simulink model "CF018A_GmRoadWhlInQlfr"  (R2013b)
settings: Solver=FixedStepDiscrete  SolverMode=SingleTasking  StartTime=0.0  StopTime=1  FixedStep=0.002  RelTol=1e-3
values from neighbouring files (symbols this model uses):
  DELTAPLSROLLOVR_CNT_S16 = DataDict.Constant    [CF018A_GmRoadWhlInQlfr_DataDict.m]
  DELTATISTAMPCNTROLLOVR_CNT_S32 = DataDict.Constant    [CF018A_GmRoadWhlInQlfr_DataDict.m]
  GmRoadWhlInQlfrMaxAllwblFrq = DataDict.Calibration    [CF018A_GmRoadWhlInQlfr_DataDict.m]
  GmRoadWhlInQlfrMaxFrqChg = DataDict.Calibration    [CF018A_GmRoadWhlInQlfr_DataDict.m]
  LEFRQCHGOUTOFRNG_CNT_U08 = DataDict.Constant    [CF018A_GmRoadWhlInQlfr_DataDict.m]
  LEFRQOUTOFRNG_CNT_U08 = DataDict.Constant    [CF018A_GmRoadWhlInQlfr_DataDict.m]
  NODEBSTEP_CNT_U16 = DataDict.Constant    [CF018A_GmRoadWhlInQlfr_DataDict.m]
  PARKDURN_CNT_F32 = DataDict.Constant    [CF018A_GmRoadWhlInQlfr_DataDict.m]
  PREVRAWWHLFRQMIN_HZ_F32 = DataDict.Constant    [CF018A_GmRoadWhlInQlfr_DataDict.m]
  RIFRQCHGOUTOFRNG_CNT_U08 = DataDict.Constant    [CF018A_GmRoadWhlInQlfr_DataDict.m]
  RIFRQOUTOFRNG_CNT_U08 = DataDict.Constant    [CF018A_GmRoadWhlInQlfr_DataDict.m]
  RoadWhlFrqInCalcOutOfRng = DataDict.NTC    [CF018A_GmRoadWhlInQlfr_DataDict.m]
  SECTO100MICROSECCNVN_CNT_F32 = DataDict.Constant    [CF018A_GmRoadWhlInQlfr_DataDict.m]
  WHLFRQMIN_HZ_F32 = DataDict.Constant    [CF018A_GmRoadWhlInQlfr_DataDict.m]
undefined symbols (not defined in the file or in its folder): NtcSts1
libraries: simulink x5, NxtrAbslt x2, NxtrLim x2
(part 4 of 5)

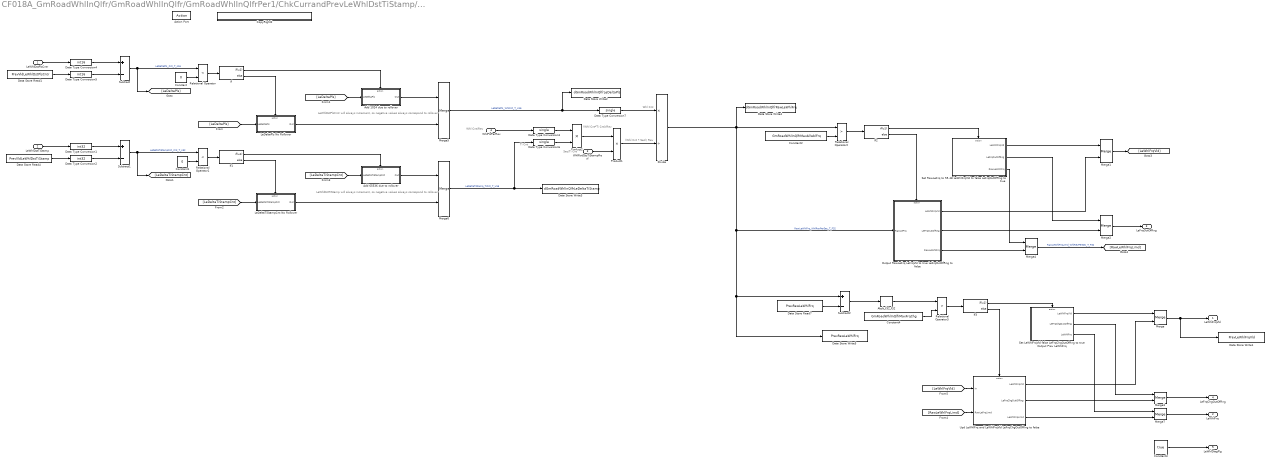
== system CF018A_GmRoadWhlInQlfr/GmRoadWhlInQlfr/GmRoadWhlInQlfrPer1/ChkCurrandPrevLeWhlDstTiStamp/Calc LeWhlFrq and LeWhlFrqVld /Calc LeWhlFrq and LeWhlFrqVld  ==
  note: Whl Cnt
  note: (Whl Cnt * Sec)/ Rev
  note: Ti Cnt
  note: Sec/Ti Cnt
  note: (Whl Cnt*Ti Cnt)/Rev
  note: Whl Cnt/Rev
  note: LeWhlDstTiStamp will always increment, so negative values always correspond to rollover
  note: LeWhlDstPlsCntr will always increment, so negative values always correspond to rollover
  LeWhlDstPlsCntr : Inport  RequirementInfo="{'linktype_rmi_doors' '0000c6e7 (/GM T1XX/SubSystem Specifications/Customer Functions/CF018A GM Road Wheel Input Qualifier)' '#170' 'true' 'REQ:  170' '' } %GIDa_81f6eb15_8b18_4642_a58d_cf70759d8f15"
  LeWhlDstTiStamp : Inport  RequirementInfo="{'linktype_rmi_doors' '0000c6e7 (/GM T1XX/SubSystem Specifications/Customer Functions/CF018A GM Road Wheel Input Qualifier)' '#170' 'true' 'REQ:  170' '' } %GIDa_7f9ec301_ef8f_4782_8c21_3364c3472735"  Port=2
  WhlRotlStsTiStampResl : Inport  RequirementInfo="{'linktype_rmi_doors' '0000c6e7 (/GM T1XX/SubSystem Specifications/Customer Functions/CF018A GM Road Wheel Input Qualifier)' '#170' 'true' 'REQ:  170' '' } %GIDa_d73dd23d_3d37_412a_b785_a9f4fffd0110"  Port=3
  WhlPlsPerRev : Inport  RequirementInfo="{'linktype_rmi_doors' '0000c6e7 (/GM T1XX/SubSystem Specifications/Customer Functions/CF018A GM Road Wheel Input Qualifier)' '#170' 'true' 'REQ:  170' '' } %GIDa_d298984b_0588_461a_81d7_4aff6f4fa4fc"  Port=4
  Action Port : ActionPort  ActionType=then
  Abslt_f32_f32 : NxtrAbslt/Abslt_f32_f32  RequirementInfo="{'linktype_rmi_doors' '0000c6e7 (/GM T1XX/SubSystem Specifications/Customer Functions/CF018A GM Road Wheel Input Qualifier)' '#176' 'true' 'REQ:  176' '' } %GIDa_9babf064_4138_43f4_bcce_3d87a0d45cc3"  SFunctionSpec=single y1 = Abslt_f32_f32(single u1)
      settings: AttributesFormatString=%<Name>
  Add 1024 due to rollover : Subsystem  RequirementInfo="{'linktype_rmi_doors' '0000c6e7 (/GM T1XX/SubSystem Specifications/Customer Functions/CF018A GM Road Wheel Input Qualifier)' '#170' 'true' 'REQ:  170' '' } %GIDa_49dd0180_17d4_41ca_993d_8e15b0be8cd1"  TreatAsAtomicUnit=on
  Add 65536 due to rollover : Subsystem  RequirementInfo="{'linktype_rmi_doors' '0000c6e7 (/GM T1XX/SubSystem Specifications/Customer Functions/CF018A GM Road Wheel Input Qualifier)' '#170' 'true' 'REQ:  170' '' } %GIDa_673682fc_2422_4a83_b510_e76deceeae94"  TreatAsAtomicUnit=on
  Constant : Constant  RequirementInfo="{'linktype_rmi_doors' '0000c6e7 (/GM T1XX/SubSystem Specifications/Customer Functions/CF018A GM Road Wheel Input Qualifier)' '#170' 'true' 'REQ:  170' '' } %GIDa_8b061d41_99c2_4522_a106_d56cc84f1816"  Value=0  OutDataTypeStr=int16
  Constant1 : Constant  RequirementInfo="{'linktype_rmi_doors' '0000c6e7 (/GM T1XX/SubSystem Specifications/Customer Functions/CF018A GM Road Wheel Input Qualifier)' '#170' 'true' 'REQ:  170' '' } %GIDa_ddec956e_1640_4ce9_b7f4_876fb629fee2"  Value=0  OutDataTypeStr=int32
  Constant2 : Constant  RequirementInfo="{'linktype_rmi_doors' '0000c6e7 (/GM T1XX/SubSystem Specifications/Customer Functions/CF018A GM Road Wheel Input Qualifier)' '#218' 'true' 'REQ:  218' '' ; 'linktype_rmi_doors' '0000c6e7 (/GM T1XX/SubSystem Specifications/Customer Functions/CF018A GM Road Wheel Input Qualifier)' '#175' 'true' 'REQ:  175' '' } %GIDa_4876d398_3911_425d_a27f_6993c3547bbd"  Value=GmRoadWhlInQlfrMaxAllwblFrq  OutDataTypeStr=single
  Constant3 : Constant  Value=true  OutDataTypeStr=boolean
      settings: AttributesFormatString=%<OutDataTypeStr>
  Constant4 : Constant  RequirementInfo="{'linktype_rmi_doors' '0000c6e7 (/GM T1XX/SubSystem Specifications/Customer Functions/CF018A GM Road Wheel Input Qualifier)' '#179' 'true' 'REQ:  179' '' ; 'linktype_rmi_doors' '0000c6e7 (/GM T1XX/SubSystem Specifications/Customer Functions/CF018A GM Road Wheel Input Qualifier)' '#176' 'true' 'REQ:  176' '' } %GIDa_f2aca31b_6717_44ff_958c_77a280e79e96"  Value=GmRoadWhlInQlfrMaxFrqChg
  CopyRight2 : Subsystem  Description=|  mask(Copyright Information){none=on}
      | Copyright info block.                                               
      |                                                                     
      | Place copyright information at the top of every subsystem in design.
      mask prompts: none "No parameters"
      mask help: Place copyright information at the top of every subsystem in design.
      mask Display:
      | NxtrConf = 'Nexteer Confidential';
      | 
      | sys = bdroot; %handle for the current model ("system")
      | first = get_param(sys,'Created');
      | if(isempty(first))
      |     first = datestr(now,'yyyy');
      | else
      |     first = first(end-3:end);  %year is last four digits
      | end
      | 
      | last = get_param(sys,'LastModifiedDate');
      | if isempty(last)
      |     last = datestr(now,'yyyy');
      | else
      |     last = last(end-3:end);
      | end
      | 
      | if strcmp(first,last)
      |     fprintf('%s -- Copyright %s Nexteer',NxtrConf,first)
      | else
      |     fprintf('%s -- %s%s- %s Nexteer',NxtrConf,char(169),first,last)
      | end
  Data Store Read1 : DataStoreRead  RequirementInfo="{'linktype_rmi_doors' '0000c6e7 (/GM T1XX/SubSystem Specifications/Customer Functions/CF018A GM Road Wheel Input Qualifier)' '#170' 'true' 'REQ:  170' '' } %GIDa_858aa324_7acc_4fd0_add3_db541b4b92e1"  DataStoreName=PrevVldLeWhlDstPlsCntr
  Data Store Read4 : DataStoreRead  RequirementInfo="{'linktype_rmi_doors' '0000c6e7 (/GM T1XX/SubSystem Specifications/Customer Functions/CF018A GM Road Wheel Input Qualifier)' '#170' 'true' 'REQ:  170' '' } %GIDa_7cd45e9a_58fd_4604_96cb_553a32710b34"  DataStoreName=PrevVldLeWhlDstTiStamp
  Data Store Read7 : DataStoreRead  RequirementInfo="{'linktype_rmi_doors' '0000c6e7 (/GM T1XX/SubSystem Specifications/Customer Functions/CF018A GM Road Wheel Input Qualifier)' '#176' 'true' 'REQ:  176' '' } %GIDa_a3115ec7_f18e_4431_ab97_984f5a4506dd"  Priority=0  DataStoreName=PrevRawLeWhlFrq
      settings: AttributesFormatString=%<Priority>
  Data Store Write1 : DataStoreWrite  RequirementInfo="{'linktype_rmi_doors' '0000c6e7 (/GM T1XX/SubSystem Specifications/Customer Functions/CF018A GM Road Wheel Input Qualifier)' '#176' 'true' 'REQ:  176' '' } %GIDa_ec08d42e_6251_41c8_b133_3f036ebc3510"  DataStoreName=PrevLeWhlFrqVld
      settings: AttributesFormatString=%<Priority>
  Data Store Write2 : DataStoreWrite  RequirementInfo="{'linktype_rmi_doors' '0000c6e7 (/GM T1XX/SubSystem Specifications/Customer Functions/CF018A GM Road Wheel Input Qualifier)' '#170' 'true' 'REQ:  170' '' } %GIDa_6506a920_d21b_4a41_8912_67910f5698ca"  DataStoreName=dGmRoadWhlInQlfrLeDeltaPls
  Data Store Write3 : DataStoreWrite  RequirementInfo="{'linktype_rmi_doors' '0000c6e7 (/GM T1XX/SubSystem Specifications/Customer Functions/CF018A GM Road Wheel Input Qualifier)' '#170' 'true' 'REQ:  170' '' } %GIDa_87548ccd_19bf_4323_b435_bb85d0142e2f"  DataStoreName=dGmRoadWhlInQlfrLeDeltaTiStamp
  Data Store Write4 : DataStoreWrite  RequirementInfo="{'linktype_rmi_doors' '0000c6e7 (/GM T1XX/SubSystem Specifications/Customer Functions/CF018A GM Road Wheel Input Qualifier)' '#175' 'true' 'REQ:  175' '' } %GIDa_013f3107_74ec_4409_b820_3123d1eae997"  DataStoreName=dGmRoadWhlInQlfrRawLeWhlFrq
  Data Store Write5 : DataStoreWrite  RequirementInfo="{'linktype_rmi_doors' '0000c6e7 (/GM T1XX/SubSystem Specifications/Customer Functions/CF018A GM Road Wheel Input Qualifier)' '#176' 'true' 'REQ:  176' '' } %GIDa_de1d07c8_712c_4036_8c18_78f028d520f4"  Priority=1  DataStoreName=PrevRawLeWhlFrq
      settings: AttributesFormatString=%<Priority>
  Data Type Conversion1 : DataTypeConversion  OutDataTypeStr=int32
  Data Type Conversion2 : DataTypeConversion  OutDataTypeStr=int32
  Data Type Conversion3 : DataTypeConversion  RequirementInfo="{'linktype_rmi_doors' '0000c6e7 (/GM T1XX/SubSystem Specifications/Customer Functions/CF018A GM Road Wheel Input Qualifier)' '#170' 'true' 'REQ:  170' '' } %GIDa_0b3a842d_d2aa_433d_8a7e_1a628cbde61e"  OutDataTypeStr=single
  Data Type Conversion4 : DataTypeConversion  OutDataTypeStr=int16
  Data Type Conversion5 : DataTypeConversion  OutDataTypeStr=int16
  Data Type Conversion6 : DataTypeConversion  RequirementInfo="{'linktype_rmi_doors' '0000c6e7 (/GM T1XX/SubSystem Specifications/Customer Functions/CF018A GM Road Wheel Input Qualifier)' '#170' 'true' 'REQ:  170' '' } %GIDa_d0f1bc26_581c_47ab_b06b_8b782c2ae32a"  OutDataTypeStr=single
  Data Type Conversion7 : DataTypeConversion  RequirementInfo="{'linktype_rmi_doors' '0000c6e7 (/GM T1XX/SubSystem Specifications/Customer Functions/CF018A GM Road Wheel Input Qualifier)' '#170' 'true' 'REQ:  170' '' } %GIDa_806b0f95_0ee7_4aef_8557_915ee92f77aa"  OutDataTypeStr=single
  Divide : Product  RequirementInfo="{'linktype_rmi_doors' '0000c6e7 (/GM T1XX/SubSystem Specifications/Customer Functions/CF018A GM Road Wheel Input Qualifier)' '#170' 'true' 'REQ:  170' '' } %GIDa_ecaab946_6f87_48de_9311_216db4035167"  Inputs=*/
      settings: AttributesFormatString=%<Priority>
  If : If  RequirementInfo="{'linktype_rmi_doors' '0000c6e7 (/GM T1XX/SubSystem Specifications/Customer Functions/CF018A GM Road Wheel Input Qualifier)' '#170' 'true' 'REQ:  170' '' } %GIDa_c1572c43_595f_4241_bfc8_833d91f05090"  IfExpression=u1
  If1 : If  RequirementInfo="{'linktype_rmi_doors' '0000c6e7 (/GM T1XX/SubSystem Specifications/Customer Functions/CF018A GM Road Wheel Input Qualifier)' '#170' 'true' 'REQ:  170' '' } %GIDa_8ea9250d_47f8_4248_b574_e8d129d6ab18"  IfExpression=u1
  If2 : If  RequirementInfo="{'linktype_rmi_doors' '0000c6e7 (/GM T1XX/SubSystem Specifications/Customer Functions/CF018A GM Road Wheel Input Qualifier)' '#175' 'true' 'REQ:  175' '' } %GIDa_3c20a0fd_f252_4d8c_93c2_0ab938042c19"  IfExpression=u1
  If3 : If  RequirementInfo="{'linktype_rmi_doors' '0000c6e7 (/GM T1XX/SubSystem Specifications/Customer Functions/CF018A GM Road Wheel Input Qualifier)' '#176' 'true' 'REQ:  176' '' } %GIDa_0bf69924_8eac_4bad_96f1_7da21f21de67"  IfExpression=u1
  LeDeltaPls No Rollover : Subsystem  RequirementInfo="{'linktype_rmi_doors' '0000c6e7 (/GM T1XX/SubSystem Specifications/Customer Functions/CF018A GM Road Wheel Input Qualifier)' '#170' 'true' 'REQ:  170' '' } %GIDa_731e1fb5_a310_441e_ab2e_f04067f21e71"  TreatAsAtomicUnit=on
  LeDeltaTiStampCnt No Rollover : Subsystem  RequirementInfo="{'linktype_rmi_doors' '0000c6e7 (/GM T1XX/SubSystem Specifications/Customer Functions/CF018A GM Road Wheel Input Qualifier)' '#170' 'true' 'REQ:  170' '' } %GIDa_baedfd9e_836e_480d_9447_1e736d4e0fac"  TreatAsAtomicUnit=on
  Merge : Merge  RequirementInfo="{'linktype_rmi_doors' '0000c6e7 (/GM T1XX/SubSystem Specifications/Customer Functions/CF018A GM Road Wheel Input Qualifier)' '#176' 'true' 'REQ:  176' '' } %GIDa_51a3869e_ea98_4a3c_8ce5_bfb21175d061"
  Merge1 : Merge  RequirementInfo="{'linktype_rmi_doors' '0000c6e7 (/GM T1XX/SubSystem Specifications/Customer Functions/CF018A GM Road Wheel Input Qualifier)' '#175' 'true' 'REQ:  175' '' } %GIDa_4ee51a38_6586_419f_8521_cb767c7b3f04"
  Merge2 : Merge  RequirementInfo="{'linktype_rmi_doors' '0000c6e7 (/GM T1XX/SubSystem Specifications/Customer Functions/CF018A GM Road Wheel Input Qualifier)' '#175' 'true' 'REQ:  175' '' } %GIDa_5e7a4cc5_3ac2_4b71_ba3d_f061c882e117"
  Merge3 : Merge  RequirementInfo="{'linktype_rmi_doors' '0000c6e7 (/GM T1XX/SubSystem Specifications/Customer Functions/CF018A GM Road Wheel Input Qualifier)' '#176' 'true' 'REQ:  176' '' } %GIDa_4213d823_ddd0_495b_8a3d_1c6b4d776feb"
  Merge4 : Merge  RequirementInfo="{'linktype_rmi_doors' '0000c6e7 (/GM T1XX/SubSystem Specifications/Customer Functions/CF018A GM Road Wheel Input Qualifier)' '#175' 'true' 'REQ:  175' '' } %GIDa_2a1d9456_a63f_4485_83e8_e75f4ada7506"
  Merge5 : Merge  RequirementInfo="{'linktype_rmi_doors' '0000c6e7 (/GM T1XX/SubSystem Specifications/Customer Functions/CF018A GM Road Wheel Input Qualifier)' '#170' 'true' 'REQ:  170' '' } %GIDa_5b3df2ac_8a4a_439d_a557_913bc624ef85"
  Merge6 : Merge  RequirementInfo="{'linktype_rmi_doors' '0000c6e7 (/GM T1XX/SubSystem Specifications/Customer Functions/CF018A GM Road Wheel Input Qualifier)' '#170' 'true' 'REQ:  170' '' } %GIDa_5feceb6f_cf07_4d53_9b7a_58b2e1e87157"
  Merge7 : Merge  RequirementInfo="{'linktype_rmi_doors' '0000c6e7 (/GM T1XX/SubSystem Specifications/Customer Functions/CF018A GM Road Wheel Input Qualifier)' '#176' 'true' 'REQ:  176' '' } %GIDa_158f11e6_aafd_45d3_bb19_68f95431a00e"
  Output RawLeFrq LeFrqVld to true LeFrqOutOfRng to false : Subsystem  RequirementInfo="{'linktype_rmi_doors' '0000c6e7 (/GM T1XX/SubSystem Specifications/Customer Functions/CF018A GM Road Wheel Input Qualifier)' '#175' 'true' 'REQ:  175' '' } %GIDa_de6b13e0_e9eb_4a05_8dff_8bfc345d5c25"  TreatAsAtomicUnit=on
  Product1 : Product  RequirementInfo="{'linktype_rmi_doors' '0000c6e7 (/GM T1XX/SubSystem Specifications/Customer Functions/CF018A GM Road Wheel Input Qualifier)' '#170' 'true' 'REQ:  170' '' } %GIDa_e290239d_3e19_4a86_aa29_128c5d82eca0"
  Product2 : Product  RequirementInfo="{'linktype_rmi_doors' '0000c6e7 (/GM T1XX/SubSystem Specifications/Customer Functions/CF018A GM Road Wheel Input Qualifier)' '#170' 'true' 'REQ:  170' '' } %GIDa_4677af3e_0b4c_43df_8a08_cd284f17272b"
  Relational Operator : RelationalOperator  RequirementInfo="{'linktype_rmi_doors' '0000c6e7 (/GM T1XX/SubSystem Specifications/Customer Functions/CF018A GM Road Wheel Input Qualifier)' '#170' 'true' 'REQ:  170' '' } %GIDa_752c2c9e_41d6_492c_850f_450902082c43"  Operator=<  OutDataTypeStr=boolean
  Relational Operator1 : RelationalOperator  RequirementInfo="{'linktype_rmi_doors' '0000c6e7 (/GM T1XX/SubSystem Specifications/Customer Functions/CF018A GM Road Wheel Input Qualifier)' '#170' 'true' 'REQ:  170' '' } %GIDa_f32f7a75_e353_422e_832d_c9335738dc5a"  Operator=<  OutDataTypeStr=boolean
  Relational Operator2 : RelationalOperator  RequirementInfo="{'linktype_rmi_doors' '0000c6e7 (/GM T1XX/SubSystem Specifications/Customer Functions/CF018A GM Road Wheel Input Qualifier)' '#175' 'true' 'REQ:  175' '' } %GIDa_a36d66af_8ed3_4599_8ceb_4e44b369b520"  Operator=>  OutDataTypeStr=boolean
  Relational Operator3 : RelationalOperator  RequirementInfo="{'linktype_rmi_doors' '0000c6e7 (/GM T1XX/SubSystem Specifications/Customer Functions/CF018A GM Road Wheel Input Qualifier)' '#176' 'true' 'REQ:  176' '' } %GIDa_280c3b32_0b0f_4faa_b9b8_ef69c1361a72"  Operator=>  OutDataTypeStr=boolean
  Set LeWhlFrqVld false LeFrqChgOutOfRng to true Output Prev LeWhlFrq : Subsystem  RequirementInfo="{'linktype_rmi_doors' '0000c6e7 (/GM T1XX/SubSystem Specifications/Customer Functions/CF018A GM Road Wheel Input Qualifier)' '#176' 'true' 'REQ:  176' '' } %GIDa_69e17394_4547_4791_9f0a_6f0549775007"  TreatAsAtomicUnit=on
  Set RawLeFrq to 55.48 LeWhlFrqVld to false LeFrqOutOfRng to true : Subsystem  RequirementInfo="{'linktype_rmi_doors' '0000c6e7 (/GM T1XX/SubSystem Specifications/Customer Functions/CF018A GM Road Wheel Input Qualifier)' '#175' 'true' 'REQ:  175' '' } %GIDa_ca636fc7_8999_459a_8a1a_72b0b121a43f"  TreatAsAtomicUnit=on
  Subtract : Sum  RequirementInfo="{'linktype_rmi_doors' '0000c6e7 (/GM T1XX/SubSystem Specifications/Customer Functions/CF018A GM Road Wheel Input Qualifier)' '#170' 'true' 'REQ:  170' '' } %GIDa_a619972a_c82a_4aa5_8379_e381c0276a01"  Inputs=+-  OutDataTypeStr=int16
      settings: AttributesFormatString=%<Priority>
  Subtract1 : Sum  RequirementInfo="{'linktype_rmi_doors' '0000c6e7 (/GM T1XX/SubSystem Specifications/Customer Functions/CF018A GM Road Wheel Input Qualifier)' '#170' 'true' 'REQ:  170' '' } %GIDa_988c2c08_2083_452e_80ea_7c9ead94b42f"  Inputs=+-  OutDataTypeStr=int32
      settings: AttributesFormatString=%<Priority>
  Subtract2 : Sum  RequirementInfo="{'linktype_rmi_doors' '0000c6e7 (/GM T1XX/SubSystem Specifications/Customer Functions/CF018A GM Road Wheel Input Qualifier)' '#176' 'true' 'REQ:  176' '' } %GIDa_824b8546_ee4a_4296_8369_853dd7941f8a"  Inputs=+-
  Upd LeWhlFrq and LeWhlFrqVld LeFrqChgOutOfRng to false : Subsystem  RequirementInfo="{'linktype_rmi_doors' '0000c6e7 (/GM T1XX/SubSystem Specifications/Customer Functions/CF018A GM Road Wheel Input Qualifier)' '#176' 'true' 'REQ:  176' '' } %GIDa_d364e30d_9bb3_46d4_87ee_ef84be4eddae"  TreatAsAtomicUnit=on
  LeWhlFrqVld : Outport  RequirementInfo="{'linktype_rmi_doors' '0000c6e7 (/GM T1XX/SubSystem Specifications/Customer Functions/CF018A GM Road Wheel Input Qualifier)' '#176' 'true' 'REQ:  176' '' } %GIDa_bf05f879_8f7d_42a0_b324_aeb1286c9553"
  LeWhlFrq : Outport  RequirementInfo="{'linktype_rmi_doors' '0000c6e7 (/GM T1XX/SubSystem Specifications/Customer Functions/CF018A GM Road Wheel Input Qualifier)' '#176' 'true' 'REQ:  176' '' } %GIDa_d83b31f1_6e5b_4863_aa9e_369246e7f69e"  Port=2
  LeFrqOutOfRng : Outport  RequirementInfo="{'linktype_rmi_doors' '0000c6e7 (/GM T1XX/SubSystem Specifications/Customer Functions/CF018A GM Road Wheel Input Qualifier)' '#175' 'true' 'REQ:  175' '' } %GIDa_69a60709_30d0_4c0e_afbd_b91f3e065487"  Port=3
  LeFrqChgOutOfRng : Outport  RequirementInfo="{'linktype_rmi_doors' '0000c6e7 (/GM T1XX/SubSystem Specifications/Customer Functions/CF018A GM Road Wheel Input Qualifier)' '#176' 'true' 'REQ:  176' '' } %GIDa_3d57b922_5289_402f_9db8_c179b75ec954"  Port=4
  LeWhlDiagFlg : Outport  Port=5
  wires:
  If/1 -> Add 1024 due to rollover/Action
  LeWhlDstPlsCntr/1 -> Data Type Conversion4/1
  Subtract/1 -> [LeDeltaPls], Relational Operator/1  "LeDeltaPls_Cnt_T_s16"
  Relational Operator/1 -> If/1
  Constant/1 -> Relational Operator/2
  If1/1 -> Add 65536 due to rollover/Action
  Subtract1/1 -> [LeDeltaTiStampCnt], Relational Operator1/1  "LeDeltaTiStampCnt_Cnt_T_s32"
  Relational Operator1/1 -> If1/1
  Constant1/1 -> Relational Operator1/2
  Constant2/1 -> Relational Operator2/2
  Relational Operator2/1 -> If2/1
  If2/1 -> Set RawLeFrq to 55.48 LeWhlFrqVld to false LeFrqOutOfRng to true/Action
  Divide/1 -> Data Store Write4/1, Relational Operator2/1, Output RawLeFrq LeFrqVld to true LeFrqOutOfRng to false/1(RawLeFrq), Subtract2/1, Data Store Write5/1  "RawLeWhlFrq_WhlRevPerSec_T_F32"
  Data Store Read7/1 -> Subtract2/2
  Constant4/1 -> Relational Operator3/2
  Relational Operator3/1 -> If3/1
  Subtract2/1 -> Abslt_f32_f32/1
  If3/1 -> Set LeWhlFrqVld false LeFrqChgOutOfRng to true Output Prev LeWhlFrq/Action
  If3/2 -> Upd LeWhlFrq and LeWhlFrqVld LeFrqChgOutOfRng to false/Action
  Upd LeWhlFrq and LeWhlFrqVld LeFrqChgOutOfRng to false/1(LeWhlFrqVld) -> Merge/2
  Set LeWhlFrqVld false LeFrqChgOutOfRng to true Output Prev LeWhlFrq/1(LeWhlFrqVld) -> Merge/1
  Merge/1 -> Data Store Write1/1, LeWhlFrqVld/1
  If2/2 -> Output RawLeFrq LeFrqVld to true LeFrqOutOfRng to false/Action
  WhlPlsPerRev/1 -> Data Type Conversion3/1
  Abslt_f32_f32/1 -> Relational Operator3/1
  WhlRotlStsTiStampResl/1 -> Product1/2
  Product1/1 -> Divide/2
  [LeDeltaPls] -> LeDeltaPls No Rollover/1(LeDeltaPls)
  [LeDeltaTiStampCnt] -> LeDeltaTiStampCnt No Rollover/1(LeDeltaTiStampCnt)
  If/2 -> LeDeltaPls No Rollover/Action
  [LeDeltaPls] -> Add 1024 due to rollover/1(LeDeltaPls)
  If1/2 -> LeDeltaTiStampCnt No Rollover/Action
  [LeDeltaTiStampCnt] -> Add 65536 due to rollover/1(LeDeltaTiStampCnt)
  Product2/1 -> Product1/1
  Data Store Read1/1 -> Data Type Conversion5/1
  Data Type Conversion7/1 -> Divide/1
  Set RawLeFrq to 55.48 LeWhlFrqVld to false LeFrqOutOfRng to true/1(LeWhlFrqVld) -> Merge1/1
  Output RawLeFrq LeFrqVld to true LeFrqOutOfRng to false/1(LeWhlFrqVld) -> Merge1/2
  Merge2/1 -> LeFrqOutOfRng/1
  Set RawLeFrq to 55.48 LeWhlFrqVld to false LeFrqOutOfRng to true/2(LeFrqOutOfRng) -> Merge2/1
  Output RawLeFrq LeFrqVld to true LeFrqOutOfRng to false/2(LeFrqOutOfRng) -> Merge2/2
  [RawLeWhlFrqLimd] -> Upd LeWhlFrq and LeWhlFrqVld LeFrqChgOutOfRng to false/2(RawLeFrqLimd)
  Merge1/1 -> [LeWhlFrqVld]
  [LeWhlFrqVld] -> Upd LeWhlFrq and LeWhlFrqVld LeFrqChgOutOfRng to false/1(In)
  Set LeWhlFrqVld false LeFrqChgOutOfRng to true Output Prev LeWhlFrq/2(LeFrqChgOutOfRng) -> Merge3/1
  Merge3/1 -> LeFrqChgOutOfRng/1
  Output RawLeFrq LeFrqVld to true LeFrqOutOfRng to false/3(RawLeWhlFrq) -> Merge4/2
  Set RawLeFrq to 55.48 LeWhlFrqVld to false LeFrqOutOfRng to true/3(RawLeWhlFrq) -> Merge4/1
  Merge4/1 -> [RawLeWhlFrqLimd]  "RawLeWhlFrqLimd_WhlRevPerSec_T_F32"
  Upd LeWhlFrq and LeWhlFrqVld LeFrqChgOutOfRng to false/2(LeFrqChgOutOfRng) -> Merge3/2
  Add 1024 due to rollover/1(Out) -> Merge5/1
  LeDeltaPls No Rollover/1(Out) -> Merge5/2
  Merge5/1 -> Data Type Conversion7/1, Data Store Write2/1  "LeDeltaPls_WhlCnt_T_U16"
  Add 65536 due to rollover/1(Out) -> Merge6/1
  LeDeltaTiStampCnt No Rollover/1(Out) -> Merge6/2
  Merge6/1 -> Data Type Conversion6/1, Data Store Write3/1  "LeDeltaTiStamp_TiCnt_T_U16"
  Constant3/1 -> LeWhlDiagFlg/1
  Merge7/1 -> LeWhlFrq/1
  Set LeWhlFrqVld false LeFrqChgOutOfRng to true Output Prev LeWhlFrq/3(LeWhlFrq) -> Merge7/1
  Upd LeWhlFrq and LeWhlFrqVld LeFrqChgOutOfRng to false/3(LeWhlFrqLimd) -> Merge7/2
  LeWhlDstTiStamp/1 -> Data Type Conversion1/1
  Data Store Read4/1 -> Data Type Conversion2/1
  Data Type Conversion2/1 -> Subtract1/2
  Data Type Conversion1/1 -> Subtract1/1
  Data Type Conversion6/1 -> Product2/2
  Data Type Conversion5/1 -> Subtract/2
  Data Type Conversion4/1 -> Subtract/1
  Data Type Conversion3/1 -> Product2/1

== system CF018A_GmRoadWhlInQlfr/GmRoadWhlInQlfr/GmRoadWhlInQlfrPer1/ChkCurrandPrevLeWhlDstTiStamp/Calc LeWhlFrq and LeWhlFrqVld /CopyRight2 ==

== system CF018A_GmRoadWhlInQlfr/GmRoadWhlInQlfr/GmRoadWhlInQlfrPer1/ChkCurrandPrevLeWhlDstTiStamp/Calc LeWhlFrq and LeWhlFrqVld /GetRefTmr100MicroSec32bit ==
  note: 1 count = 100 uSec
  note: seconds
  note: microseconds
  note: counts
  note: Wrap-to-zero
  note: GetRefTmr100MicroSec32bit
  note: Created Aug 18, 2015
      | Modified Oct 21, 2015
      | Modified Oct 30, 2015
      | Kevin Derry
  CopyRight2 : Subsystem  Description=|  mask(Copyright Information){none=on}
      | Copyright info block.                                               
      |                                                                     
      | Place copyright information at the top of every subsystem in design.
      mask prompts: none "No parameters"
      mask help: Place copyright information at the top of every subsystem in design.
      mask Display:
      | NxtrConf = 'Nexteer Confidential';
      | 
      | sys = bdroot; %handle for the current model ("system")
      | first = get_param(sys,'Created');
      | if(isempty(first))
      |     first = datestr(now,'yyyy');
      | else
      |     first = first(end-3:end);  %year is last four digits
      | end
      | 
      | last = get_param(sys,'LastModifiedDate');
      | if isempty(last)
      |     last = datestr(now,'yyyy');
      | else
      |     last = last(end-3:end);
      | end
      | 
      | if strcmp(first,last)
      |     fprintf('%s -- Copyright %s Nexteer',NxtrConf,first)
      | else
      |     fprintf('%s -- %s%s- %s Nexteer',NxtrConf,char(169),first,last)
      | end
  Count per uSec : Constant  Value=0.01
  Data Store Read1 : DataStoreRead  DataStoreName=SimnTi
  Data Type Conversion1 : DataTypeConversion  OutDataTypeStr=uint32
  Divide1 : Product  Inputs=**
  Divide2 : Product  Inputs=*/
  Max Counts : Constant  Value=2^32-1
  Product1 : Product
  Product2 : Product
  Rounding : Rounding
  Subtract1 : Sum  Inputs=+-
  uSec per Sec : Constant  Value=1000000
  RefTmr : Outport
  wires:
  Product2/1 -> Subtract1/2
  Subtract1/1 -> Data Type Conversion1/1
  Rounding/1 -> Product2/1
  Divide2/1 -> Rounding/1
  Max Counts/1 -> Divide2/2, Product2/2
  Divide1/1 -> Divide2/1, Subtract1/1
  Product1/1 -> Divide1/1
  Count per uSec/1 -> Divide1/2
  uSec per Sec/1 -> Product1/2
  Data Type Conversion1/1 -> RefTmr/1
  Data Store Read1/1 -> Product1/1

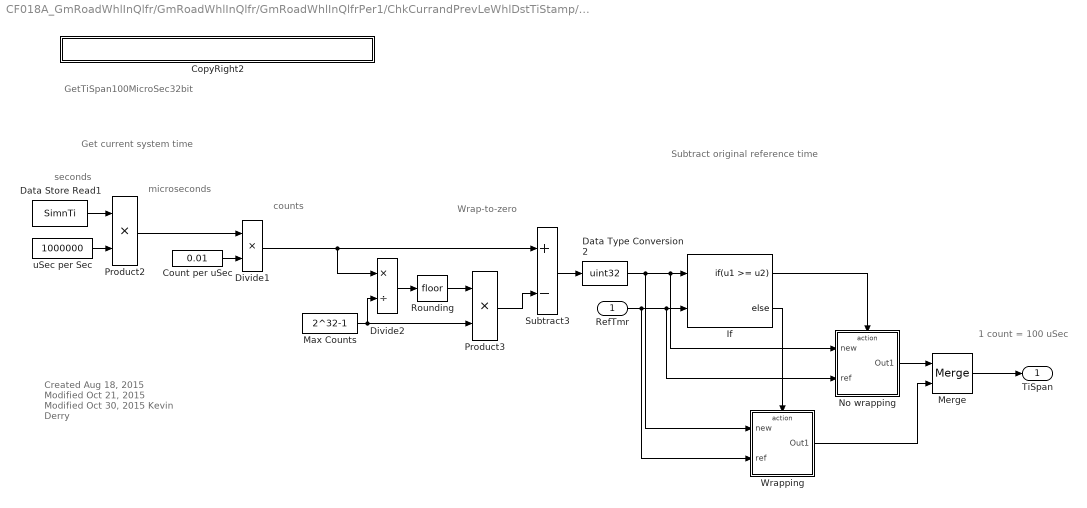
== system CF018A_GmRoadWhlInQlfr/GmRoadWhlInQlfr/GmRoadWhlInQlfrPer1/ChkCurrandPrevLeWhlDstTiStamp/Calc LeWhlFrq and LeWhlFrqVld /GetTiSpan100MicroSec32bit ==
  note: Created Aug 18, 2015
      | Modified Oct 21, 2015
      | Modified Oct 30, 2015
      | Kevin Derry
  note: GetTiSpan100MicroSec32bit
  note: Get current system time
  note: 1 count = 100 uSec
  note: Wrap-to-zero
  note: counts
  note: microseconds
  note: seconds
  note: Subtract original reference time
  RefTmr : Inport
  CopyRight2 : Subsystem  Description=|  mask(Copyright Information){none=on}
      | Copyright info block.                                               
      |                                                                     
      | Place copyright information at the top of every subsystem in design.
      mask prompts: none "No parameters"
      mask help: Place copyright information at the top of every subsystem in design.
      mask Display:
      | NxtrConf = 'Nexteer Confidential';
      | 
      | sys = bdroot; %handle for the current model ("system")
      | first = get_param(sys,'Created');
      | if(isempty(first))
      |     first = datestr(now,'yyyy');
      | else
      |     first = first(end-3:end);  %year is last four digits
      | end
      | 
      | last = get_param(sys,'LastModifiedDate');
      | if isempty(last)
      |     last = datestr(now,'yyyy');
      | else
      |     last = last(end-3:end);
      | end
      | 
      | if strcmp(first,last)
      |     fprintf('%s -- Copyright %s Nexteer',NxtrConf,first)
      | else
      |     fprintf('%s -- %s%s- %s Nexteer',NxtrConf,char(169),first,last)
      | end
  Count per uSec : Constant  Value=0.01
  Data Store Read1 : DataStoreRead  DataStoreName=SimnTi
  Data Type Conversion2 : DataTypeConversion  OutDataTypeStr=uint32
  Divide1 : Product  Inputs=**
  Divide2 : Product  Inputs=*/
  If : If  NumInputs=2  IfExpression=u1 >= u2
  Max Counts : Constant  Value=2^32-1
  Merge : Merge
  No wrapping : Subsystem  TreatAsAtomicUnit=on
  Product2 : Product
  Product3 : Product
  Rounding : Rounding
  Subtract3 : Sum  Inputs=+-
  Wrapping : Subsystem  TreatAsAtomicUnit=on
  uSec per Sec : Constant  Value=1000000
  TiSpan : Outport
  wires:
  Data Type Conversion2/1 -> Wrapping/1(new), No wrapping/1(new), If/1
  RefTmr/1 -> Wrapping/2(ref), No wrapping/2(ref), If/2
  Merge/1 -> TiSpan/1
  uSec per Sec/1 -> Product2/2
  Count per uSec/1 -> Divide1/2
  Data Store Read1/1 -> Product2/1
  Product2/1 -> Divide1/1
  Divide1/1 -> Subtract3/1, Divide2/1
  Max Counts/1 -> Product3/2, Divide2/2
  Divide2/1 -> Rounding/1
  Rounding/1 -> Product3/1
  Subtract3/1 -> Data Type Conversion2/1
  Product3/1 -> Subtract3/2
  If/1 -> No wrapping/Action
  If/2 -> Wrapping/Action
  No wrapping/1(Out1) -> Merge/1
  Wrapping/1(Out1) -> Merge/2

== system CF018A_GmRoadWhlInQlfr/GmRoadWhlInQlfr/GmRoadWhlInQlfrPer1/ChkCurrandPrevLeWhlDstTiStamp/Calc LeWhlFrq and LeWhlFrqVld /Prev LeWhlFrq and LeWhlFrqVld LeFrqOutOfRng to false LeFrqChgOutOfRng to false LeWhlDiagFlg to false  ==
  Action Port : ActionPort  ActionType=else
  Constant1 : Constant  Value=false  OutDataTypeStr=boolean
      settings: AttributesFormatString=%<OutDataTypeStr>
  Constant2 : Constant  Value=false  OutDataTypeStr=boolean
      settings: AttributesFormatString=%<OutDataTypeStr>
  Constant3 : Constant  Value=false  OutDataTypeStr=boolean
      settings: AttributesFormatString=%<OutDataTypeStr>
  CopyRight2 : Subsystem  Description=|  mask(Copyright Information){none=on}
      | Copyright info block.                                               
      |                                                                     
      | Place copyright information at the top of every subsystem in design.
      mask prompts: none "No parameters"
      mask help: Place copyright information at the top of every subsystem in design.
      mask Display:
      | NxtrConf = 'Nexteer Confidential';
      | 
      | sys = bdroot; %handle for the current model ("system")
      | first = get_param(sys,'Created');
      | if(isempty(first))
      |     first = datestr(now,'yyyy');
      | else
      |     first = first(end-3:end);  %year is last four digits
      | end
      | 
      | last = get_param(sys,'LastModifiedDate');
      | if isempty(last)
      |     last = datestr(now,'yyyy');
      | else
      |     last = last(end-3:end);
      | end
      | 
      | if strcmp(first,last)
      |     fprintf('%s -- Copyright %s Nexteer',NxtrConf,first)
      | else
      |     fprintf('%s -- %s%s- %s Nexteer',NxtrConf,char(169),first,last)
      | end
  Data Store Read2 : DataStoreRead  DataStoreName=PrevLeWhlFrqVld
      settings: AttributesFormatString=%<Priority>
  Data Store Read3 : DataStoreRead  DataStoreName=PrevLeWhlFrq
      settings: AttributesFormatString=%<Priority>
  LeWhlFrqVld : Outport
  LeWhlFrq : Outport  Port=2
  LeFrqOutOfRng : Outport  Port=3
  LeFrqChgOutOfRng : Outport  Port=4
  LeWhlDiagFlg : Outport  Port=5
  wires:
  Constant1/1 -> LeFrqOutOfRng/1
  Constant2/1 -> LeFrqChgOutOfRng/1
  Data Store Read2/1 -> LeWhlFrqVld/1
  Data Store Read3/1 -> LeWhlFrq/1
  Constant3/1 -> LeWhlDiagFlg/1

== system CF018A_GmRoadWhlInQlfr/GmRoadWhlInQlfr/GmRoadWhlInQlfrPer1/ChkCurrandPrevLeWhlDstTiStamp/Prev LeWhlFrq and LeWhlFrqVld LeFrqOutOfRng to false LeFrqChgOutOfRng to fasse LeWhlDiagFlg to false /CopyRight2 ==

== system CF018A_GmRoadWhlInQlfr/GmRoadWhlInQlfr/GmRoadWhlInQlfrPer1/NTC Diag/NTC 0x0E3 Faild/Bit0Sts fail ==
  Action Port : ActionPort  ActionType=then
  Constant : Constant  Value=LEFRQOUTOFRNG_CNT_U08
  CopyRight2 : Subsystem  Description=|  mask(Copyright Information){none=on}
      | Copyright info block.                                               
      |                                                                     
      | Place copyright information at the top of every subsystem in design.
      mask prompts: none "No parameters"
      mask help: Place copyright information at the top of every subsystem in design.
      mask Display:
      | NxtrConf = 'Nexteer Confidential';
      | 
      | sys = bdroot; %handle for the current model ("system")
      | first = get_param(sys,'Created');
      | if(isempty(first))
      |     first = datestr(now,'yyyy');
      | else
      |     first = first(end-3:end);  %year is last four digits
      | end
      | 
      | last = get_param(sys,'LastModifiedDate');
      | if isempty(last)
      |     last = datestr(now,'yyyy');
      | else
      |     last = last(end-3:end);
      | end
      | 
      | if strcmp(first,last)
      |     fprintf('%s -- Copyright %s Nexteer',NxtrConf,first)
      | else
      |     fprintf('%s -- %s%s- %s Nexteer',NxtrConf,char(169),first,last)
      | end
  Bit0Sts : Outport
  wires:
  Constant/1 -> Bit0Sts/1

== system CF018A_GmRoadWhlInQlfr/GmRoadWhlInQlfr/GmRoadWhlInQlfrPer1/NTC Diag/NTC 0x0E3 Faild/Bit0Sts pass ==
  Action Port : ActionPort  ActionType=else
  Constant1 : Constant  Value=0  OutDataTypeStr=uint8
      settings: AttributesFormatString=%<OutDataTypeStr>
  CopyRight2 : Subsystem  Description=|  mask(Copyright Information){none=on}
      | Copyright info block.                                               
      |                                                                     
      | Place copyright information at the top of every subsystem in design.
      mask prompts: none "No parameters"
      mask help: Place copyright information at the top of every subsystem in design.
      mask Display:
      | NxtrConf = 'Nexteer Confidential';
      | 
      | sys = bdroot; %handle for the current model ("system")
      | first = get_param(sys,'Created');
      | if(isempty(first))
      |     first = datestr(now,'yyyy');
      | else
      |     first = first(end-3:end);  %year is last four digits
      | end
      | 
      | last = get_param(sys,'LastModifiedDate');
      | if isempty(last)
      |     last = datestr(now,'yyyy');
      | else
      |     last = last(end-3:end);
      | end
      | 
      | if strcmp(first,last)
      |     fprintf('%s -- Copyright %s Nexteer',NxtrConf,first)
      | else
      |     fprintf('%s -- %s%s- %s Nexteer',NxtrConf,char(169),first,last)
      | end
  Bit0Sts : Outport
  wires:
  Constant1/1 -> Bit0Sts/1

== system CF018A_GmRoadWhlInQlfr/GmRoadWhlInQlfr/GmRoadWhlInQlfrPer1/NTC Diag/NTC 0x0E3 Faild/Bit1Sts fail ==
  Action Port : ActionPort  ActionType=then
  Constant : Constant  Value=LEFRQCHGOUTOFRNG_CNT_U08
  CopyRight2 : Subsystem  Description=|  mask(Copyright Information){none=on}
      | Copyright info block.                                               
      |                                                                     
      | Place copyright information at the top of every subsystem in design.
      mask prompts: none "No parameters"
      mask help: Place copyright information at the top of every subsystem in design.
      mask Display:
      | NxtrConf = 'Nexteer Confidential';
      | 
      | sys = bdroot; %handle for the current model ("system")
      | first = get_param(sys,'Created');
      | if(isempty(first))
      |     first = datestr(now,'yyyy');
      | else
      |     first = first(end-3:end);  %year is last four digits
      | end
      | 
      | last = get_param(sys,'LastModifiedDate');
      | if isempty(last)
      |     last = datestr(now,'yyyy');
      | else
      |     last = last(end-3:end);
      | end
      | 
      | if strcmp(first,last)
      |     fprintf('%s -- Copyright %s Nexteer',NxtrConf,first)
      | else
      |     fprintf('%s -- %s%s- %s Nexteer',NxtrConf,char(169),first,last)
      | end
  Bit1Sts : Outport
  wires:
  Constant/1 -> Bit1Sts/1

== system CF018A_GmRoadWhlInQlfr/GmRoadWhlInQlfr/GmRoadWhlInQlfrPer1/NTC Diag/NTC 0x0E3 Faild/Bit1Sts pass ==
  Action Port : ActionPort  ActionType=else
  Constant1 : Constant  Value=0  OutDataTypeStr=uint8
      settings: AttributesFormatString=%<OutDataTypeStr>
  CopyRight2 : Subsystem  Description=|  mask(Copyright Information){none=on}
      | Copyright info block.                                               
      |                                                                     
      | Place copyright information at the top of every subsystem in design.
      mask prompts: none "No parameters"
      mask help: Place copyright information at the top of every subsystem in design.
      mask Display:
      | NxtrConf = 'Nexteer Confidential';
      | 
      | sys = bdroot; %handle for the current model ("system")
      | first = get_param(sys,'Created');
      | if(isempty(first))
      |     first = datestr(now,'yyyy');
      | else
      |     first = first(end-3:end);  %year is last four digits
      | end
      | 
      | last = get_param(sys,'LastModifiedDate');
      | if isempty(last)
      |     last = datestr(now,'yyyy');
      | else
      |     last = last(end-3:end);
      | end
      | 
      | if strcmp(first,last)
      |     fprintf('%s -- Copyright %s Nexteer',NxtrConf,first)
      | else
      |     fprintf('%s -- %s%s- %s Nexteer',NxtrConf,char(169),first,last)
      | end
  Bit1Sts : Outport
  wires:
  Constant1/1 -> Bit1Sts/1

== system CF018A_GmRoadWhlInQlfr/GmRoadWhlInQlfr/GmRoadWhlInQlfrPer1/NTC Diag/NTC 0x0E3 Faild/Bit4Sts fail ==
  Action Port : ActionPort  ActionType=then
  Constant : Constant  Value=RIFRQOUTOFRNG_CNT_U08
  CopyRight2 : Subsystem  Description=|  mask(Copyright Information){none=on}
      | Copyright info block.                                               
      |                                                                     
      | Place copyright information at the top of every subsystem in design.
      mask prompts: none "No parameters"
      mask help: Place copyright information at the top of every subsystem in design.
      mask Display:
      | NxtrConf = 'Nexteer Confidential';
      | 
      | sys = bdroot; %handle for the current model ("system")
      | first = get_param(sys,'Created');
      | if(isempty(first))
      |     first = datestr(now,'yyyy');
      | else
      |     first = first(end-3:end);  %year is last four digits
      | end
      | 
      | last = get_param(sys,'LastModifiedDate');
      | if isempty(last)
      |     last = datestr(now,'yyyy');
      | else
      |     last = last(end-3:end);
      | end
      | 
      | if strcmp(first,last)
      |     fprintf('%s -- Copyright %s Nexteer',NxtrConf,first)
      | else
      |     fprintf('%s -- %s%s- %s Nexteer',NxtrConf,char(169),first,last)
      | end
  Bit0Sts : Outport
  wires:
  Constant/1 -> Bit0Sts/1

== system CF018A_GmRoadWhlInQlfr/GmRoadWhlInQlfr/GmRoadWhlInQlfrPer1/NTC Diag/NTC 0x0E3 Faild/Bit4Sts pass ==
  Action Port : ActionPort  ActionType=else
  Constant1 : Constant  Value=0  OutDataTypeStr=uint8
      settings: AttributesFormatString=%<OutDataTypeStr>
  CopyRight2 : Subsystem  Description=|  mask(Copyright Information){none=on}
      | Copyright info block.                                               
      |                                                                     
      | Place copyright information at the top of every subsystem in design.
      mask prompts: none "No parameters"
      mask help: Place copyright information at the top of every subsystem in design.
      mask Display:
      | NxtrConf = 'Nexteer Confidential';
      | 
      | sys = bdroot; %handle for the current model ("system")
      | first = get_param(sys,'Created');
      | if(isempty(first))
      |     first = datestr(now,'yyyy');
      | else
      |     first = first(end-3:end);  %year is last four digits
      | end
      | 
      | last = get_param(sys,'LastModifiedDate');
      | if isempty(last)
      |     last = datestr(now,'yyyy');
      | else
      |     last = last(end-3:end);
      | end
      | 
      | if strcmp(first,last)
      |     fprintf('%s -- Copyright %s Nexteer',NxtrConf,first)
      | else
      |     fprintf('%s -- %s%s- %s Nexteer',NxtrConf,char(169),first,last)
      | end
  Bit0Sts1 : Outport
  wires:
  Constant1/1 -> Bit0Sts1/1

== system CF018A_GmRoadWhlInQlfr/GmRoadWhlInQlfr/GmRoadWhlInQlfrPer1/NTC Diag/NTC 0x0E3 Faild/Bit5Sts fail ==
  Action Port : ActionPort  ActionType=then
  Constant : Constant  Value=RIFRQCHGOUTOFRNG_CNT_U08
  CopyRight2 : Subsystem  Description=|  mask(Copyright Information){none=on}
      | Copyright info block.                                               
      |                                                                     
      | Place copyright information at the top of every subsystem in design.
      mask prompts: none "No parameters"
      mask help: Place copyright information at the top of every subsystem in design.
      mask Display:
      | NxtrConf = 'Nexteer Confidential';
      | 
      | sys = bdroot; %handle for the current model ("system")
      | first = get_param(sys,'Created');
      | if(isempty(first))
      |     first = datestr(now,'yyyy');
      | else
      |     first = first(end-3:end);  %year is last four digits
      | end
      | 
      | last = get_param(sys,'LastModifiedDate');
      | if isempty(last)
      |     last = datestr(now,'yyyy');
      | else
      |     last = last(end-3:end);
      | end
      | 
      | if strcmp(first,last)
      |     fprintf('%s -- Copyright %s Nexteer',NxtrConf,first)
      | else
      |     fprintf('%s -- %s%s- %s Nexteer',NxtrConf,char(169),first,last)
      | end
  Bit1Sts : Outport
  wires:
  Constant/1 -> Bit1Sts/1

== system CF018A_GmRoadWhlInQlfr/GmRoadWhlInQlfr/GmRoadWhlInQlfrPer1/NTC Diag/NTC 0x0E3 Faild/Bit5Sts pass ==
  Action Port : ActionPort  ActionType=else
  Constant1 : Constant  Value=0  OutDataTypeStr=uint8
      settings: AttributesFormatString=%<OutDataTypeStr>
  CopyRight2 : Subsystem  Description=|  mask(Copyright Information){none=on}
      | Copyright info block.                                               
      |                                                                     
      | Place copyright information at the top of every subsystem in design.
      mask prompts: none "No parameters"
      mask help: Place copyright information at the top of every subsystem in design.
      mask Display:
      | NxtrConf = 'Nexteer Confidential';
      | 
      | sys = bdroot; %handle for the current model ("system")
      | first = get_param(sys,'Created');
      | if(isempty(first))
      |     first = datestr(now,'yyyy');
      | else
      |     first = first(end-3:end);  %year is last four digits
      | end
      | 
      | last = get_param(sys,'LastModifiedDate');
      | if isempty(last)
      |     last = datestr(now,'yyyy');
      | else
      |     last = last(end-3:end);
      | end
      | 
      | if strcmp(first,last)
      |     fprintf('%s -- Copyright %s Nexteer',NxtrConf,first)
      | else
      |     fprintf('%s -- %s%s- %s Nexteer',NxtrConf,char(169),first,last)
      | end
  Bit1Sts : Outport
  wires:
  Constant1/1 -> Bit1Sts/1

== system CF018A_GmRoadWhlInQlfr/GmRoadWhlInQlfr/GmRoadWhlInQlfrPer1/NTC Diag/NTC 0x0E3 Faild/CopyRight2 ==

== system CF018A_GmRoadWhlInQlfr/GmRoadWhlInQlfr/GmRoadWhlInQlfrPer1/NTC Diag/NTC 0x0E3 Faild/NTC 0x0E3 ==
  NtcNr : Inport
  NtcStInfo : Inport  Port=2
  NtcSts : Inport  Port=3
  DebStep : Inport  Port=4
  SetNtcSts : Subsystem  RequirementInfo={} %GIDa_1ce8ff2a_f442_4263_9752_e1c2d352aa2a  TreatAsAtomicUnit=on
      settings: RTWSystemCode=Inline
  wires:
  NtcNr/1 -> SetNtcSts/1(NtcNr)  "NtcNr"
  NtcSts/1 -> SetNtcSts/3(NtcSts)
  DebStep/1 -> SetNtcSts/4(DebStep)
  NtcStInfo/1 -> SetNtcSts/2(NtcStInfo)

== system CF018A_GmRoadWhlInQlfr/GmRoadWhlInQlfr/GmRoadWhlInQlfrPer1/NTC Diag/NTC 0x0E3 Passd/SetNtcSts ==
  NtcNr : Inport
  NtcStInfo : Inport  Port=2
  NtcSts : Inport  Port=3
  DebStep : Inport  Port=4
  CopyRight2 : Subsystem  Description=|  mask(Copyright Information){none=on}
      | Copyright info block.                                               
      |                                                                     
      | Place copyright information at the top of every subsystem in design.
      mask prompts: none "No parameters"
      mask help: Place copyright information at the top of every subsystem in design.
      mask Display:
      | NxtrConf = 'Nexteer Confidential';
      | 
      | sys = bdroot; %handle for the current model ("system")
      | first = get_param(sys,'Created');
      | first = first(end-3:end);  %year is last four digits
      | 
      | last = get_param(sys,'LastModifiedDate');
      | if isempty(last)
      |     last = datestr(now,'yyyy');
      | else
      |     last = last(end-3:end);
      | end
      | 
      | if strcmp(first,last)
      |     fprintf('%s -- Copyright %s Nexteer',NxtrConf,first)
      | else
      |     fprintf('%s -- %s%s- %s Nexteer',NxtrConf,char(169),first,last)
      | end
  Data Store Write3 : DataStoreWrite  DataStoreName=RoadWhlFrqInCalcOutOfRng
  Terminator : Terminator
  Terminator1 : Terminator
  Terminator2 : Terminator
  wires:
  DebStep/1 -> Terminator2/1
  NtcSts/1 -> Data Store Write3/1
  NtcNr/1 -> Terminator/1
  NtcStInfo/1 -> Terminator1/1

== system CF018A_GmRoadWhlInQlfr/GmRoadWhlInQlfr/GmRoadWhlInQlfrPer1/Chk Curr and Prev RiWhlDstTiStamp/Calc RiWhlFrq and RiWhlFrqVld /Calc RiWhlFrq and RiWhlFrqVld /Add 1024 due to rollover ==
  RiDeltaPls : Inport
  Action Port : ActionPort  ActionType=then
  Constant : Constant  Value=DELTAPLSROLLOVR_CNT_S16
  CopyRight2 : Subsystem  Description=|  mask(Copyright Information){none=on}
      | Copyright info block.                                               
      |                                                                     
      | Place copyright information at the top of every subsystem in design.
      mask prompts: none "No parameters"
      mask help: Place copyright information at the top of every subsystem in design.
      mask Display:
      | NxtrConf = 'Nexteer Confidential';
      | 
      | sys = bdroot; %handle for the current model ("system")
      | first = get_param(sys,'Created');
      | if(isempty(first))
      |     first = datestr(now,'yyyy');
      | else
      |     first = first(end-3:end);  %year is last four digits
      | end
      | 
      | last = get_param(sys,'LastModifiedDate');
      | if isempty(last)
      |     last = datestr(now,'yyyy');
      | else
      |     last = last(end-3:end);
      | end
      | 
      | if strcmp(first,last)
      |     fprintf('%s -- Copyright %s Nexteer',NxtrConf,first)
      | else
      |     fprintf('%s -- %s%s- %s Nexteer',NxtrConf,char(169),first,last)
      | end
  Data Type Conversion1 : DataTypeConversion  OutDataTypeStr=uint16
  Subtract : Sum  OutDataTypeStr=uint16
  Out : Outport
  wires:
  Constant/1 -> Subtract/2
  Subtract/1 -> Data Type Conversion1/1
  RiDeltaPls/1 -> Subtract/1
  Data Type Conversion1/1 -> Out/1

== system CF018A_GmRoadWhlInQlfr/GmRoadWhlInQlfr/GmRoadWhlInQlfrPer1/Chk Curr and Prev RiWhlDstTiStamp/Calc RiWhlFrq and RiWhlFrqVld /Calc RiWhlFrq and RiWhlFrqVld /Add 65536 due to rollover ==
  RiDeltaTiStampCnt : Inport
  Action Port : ActionPort  ActionType=then
  Constant : Constant  Value=DELTATISTAMPCNTROLLOVR_CNT_S32
  CopyRight2 : Subsystem  Description=|  mask(Copyright Information){none=on}
      | Copyright info block.                                               
      |                                                                     
      | Place copyright information at the top of every subsystem in design.
      mask prompts: none "No parameters"
      mask help: Place copyright information at the top of every subsystem in design.
      mask Display:
      | NxtrConf = 'Nexteer Confidential';
      | 
      | sys = bdroot; %handle for the current model ("system")
      | first = get_param(sys,'Created');
      | if(isempty(first))
      |     first = datestr(now,'yyyy');
      | else
      |     first = first(end-3:end);  %year is last four digits
      | end
      | 
      | last = get_param(sys,'LastModifiedDate');
      | if isempty(last)
      |     last = datestr(now,'yyyy');
      | else
      |     last = last(end-3:end);
      | end
      | 
      | if strcmp(first,last)
      |     fprintf('%s -- Copyright %s Nexteer',NxtrConf,first)
      | else
      |     fprintf('%s -- %s%s- %s Nexteer',NxtrConf,char(169),first,last)
      | end
  Data Type Conversion1 : DataTypeConversion  OutDataTypeStr=uint16
  Subtract : Sum  OutDataTypeStr=uint16
  Out : Outport
  wires:
  Constant/1 -> Subtract/2
  Subtract/1 -> Data Type Conversion1/1
  RiDeltaTiStampCnt/1 -> Subtract/1
  Data Type Conversion1/1 -> Out/1

== system CF018A_GmRoadWhlInQlfr/GmRoadWhlInQlfr/GmRoadWhlInQlfrPer1/Chk Curr and Prev RiWhlDstTiStamp/Calc RiWhlFrq and RiWhlFrqVld /Calc RiWhlFrq and RiWhlFrqVld /CopyRight2 ==
